simulink model "ProblemStatement1_Demodulation"  (R2021a)
settings: Solver=VariableStepAuto  StartTime=0.0  StopTime=10.0  RelTol=1e-3
settings Model: Creator=psadh  LastModifiedBy=psadh

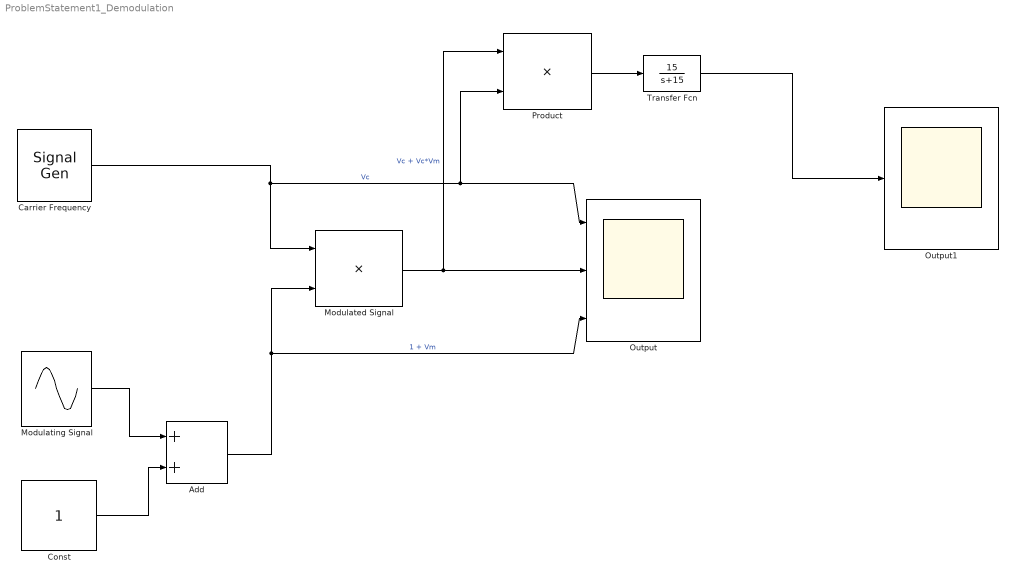
== system ProblemStatement1_Demodulation ==
  Add : Sum
  Carrier Frequency : SignalGenerator  Frequency=2*pi*4500  Units=rad/sec
  Const : Constant
  Modulated Signal : Product
  Modulating Signal : Sin  Amplitude=0.5  Frequency=2*pi*100  SampleTime=0
  Output : Scope  NumInputPorts=3
  Output1 : Scope
  Product : Product
  Transfer Fcn : TransferFcn  Numerator=[15]  Denominator=[1 15]
  wires:
  Modulating Signal/1 -> Add/1
  Const/1 -> Add/2
  Carrier Frequency/1 -> Modulated Signal/1, Product/2, Output/1  "Vc"
  Add/1 -> Modulated Signal/2, Output/3  "1 + Vm"
  Modulated Signal/1 -> Product/1, Output/2  "Vc + Vc*Vm"
  Product/1 -> Transfer Fcn/1
  Transfer Fcn/1 -> Output1/1
